simulink model "linear_system"  (R2021b)
settings: Solver=VariableStepAuto  StartTime=0.0  StopTime=10.0  RelTol=1e-8
values from neighbouring files (symbols this model uses):
  A = [ ... (first row only)    [linearized_model.m]
  B = [0; 0; c*F/E; b*F/E]    [linearized_model.m]
  C = [ ... (first row only)    [linearized_model.m]
  D = [0; 0]    [linearized_model.m]
undefined symbols (not defined in the file or in its folder): K
libraries: simulink_extras x2, simulink x2
settings Model: Creator=viking  LastModifiedBy=viking
settings SolverCC: ZeroCrossAlgorithm=Adaptive
settings DebuggingCC: UnconnectedInputMsg=none  UnconnectedOutputMsg=none  UnconnectedLineMsg=none
settings ModelReferenceCC: EnableRefExpFcnMdlSchedulingChecks=off
settings RTWCC: DLArmComputeVersion=20.02.1

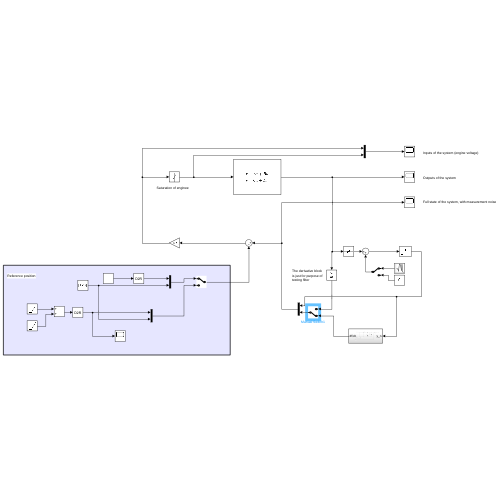
[thumbnail: Simulink's stored preview of the top-level diagram]
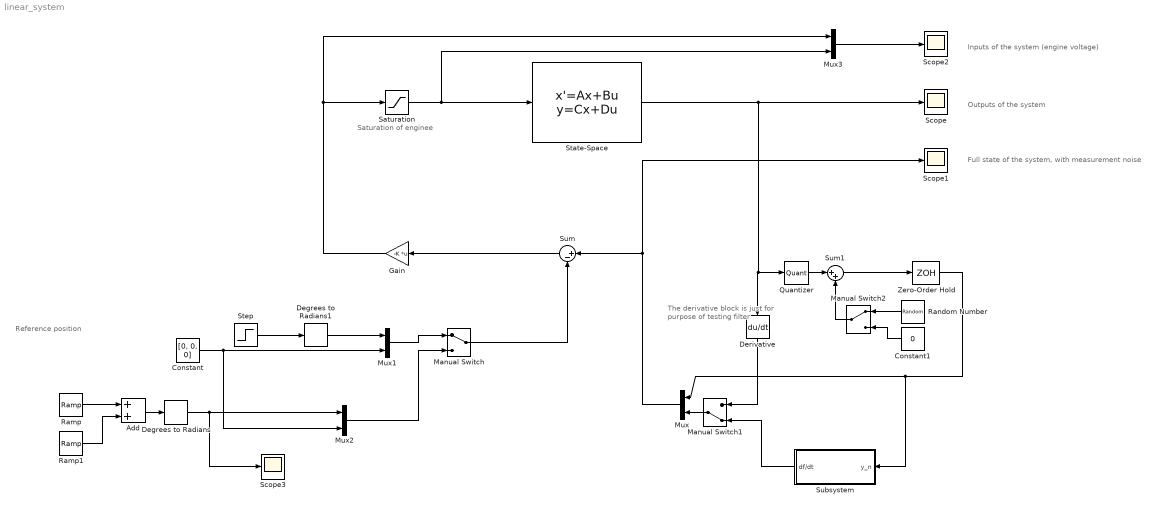
== system linear_system ==
  note: The derivative block is just for purpose of testing filter
  note: Inputs of the system (engine voltage)
  note: Full state of the system, with measurement noise
  note: Outputs of the system
  note: Saturation of enginee
  note: Reference position
  Add : Sum
  Constant : Constant  Value=[0, 0, 0]
  Constant1 : Constant  Value=0
  Degrees to Radians : simulink_extras/Transformations/Degrees to Radians
  Degrees to Radians1 : simulink_extras/Transformations/Degrees to Radians
  Derivative : Derivative  CoefficientInTFapproximation=0
  Gain : Gain  Gain=-K  Multiplication=Matrix(K*u)
  Manual Switch : ManualSwitch
  Manual Switch1 : ManualSwitch  CurrentSetting=0
  Manual Switch2 : ManualSwitch
  Mux{,1..3} (4 alike) : Mux  Inputs=2
  Quantizer : Quantizer  QuantizationInterval=0.005
  Ramp : simulink/Sources/Ramp  slope=5  start=0  InitialOutput=0
  Ramp1 : simulink/Sources/Ramp  slope=-5  start=5  InitialOutput=0
  Random Number : RandomNumber  Variance=1e-5  SampleTime=0.005
  Saturation : Saturate  UpperLimit=5  LowerLimit=-5
  Scope{,1..3} (4 alike) : Scope
  State-Space : StateSpace  A=A  B=B  C=C  D=D  InitialCondition=[0, 0, 0, 0]  ContinuousStateAttributes={'theta', 'alpha', 'dtheta', 'dalpha'}
  Step : Step  Time=0.1  After=45  SampleTime=0
  Subsystem : Subsystem
  Sum : Sum  Inputs=|+-
  Sum1 : Sum  Inputs=|++
  Zero-Order Hold : ZeroOrderHold  SampleTime=0.005
  wires:
  State-Space/1 -> Quantizer/1, Derivative/1, Scope/1
  Gain/1 -> Mux3/1, Saturation/1
  Mux/1 -> Sum/1, Scope1/1
  Sum/1 -> Gain/1
  Manual Switch/1 -> Sum/2
  Mux1/1 -> Manual Switch/1
  Constant/1 -> Mux2/2, Mux1/2
  Mux2/1 -> Manual Switch/2
  Ramp/1 -> Add/1
  Ramp1/1 -> Add/2
  Saturation/1 -> Mux3/2, State-Space/1
  Derivative/1 -> Manual Switch1/1
  Manual Switch1/1 -> Mux/2
  Subsystem/1(df/dt) -> Manual Switch1/2
  Degrees to Radians1/1 -> Mux1/1
  Step/1 -> Degrees to Radians1/1
  Add/1 -> Degrees to Radians/1
  Degrees to Radians/1 -> Scope3/1, Mux2/1
  Sum1/1 -> Zero-Order Hold/1
  Mux3/1 -> Scope2/1
  Quantizer/1 -> Sum1/1
  Zero-Order Hold/1 -> Subsystem/1(y_n), Mux/1
  Manual Switch2/1 -> Sum1/2
  Random Number/1 -> Manual Switch2/1
  Constant1/1 -> Manual Switch2/2

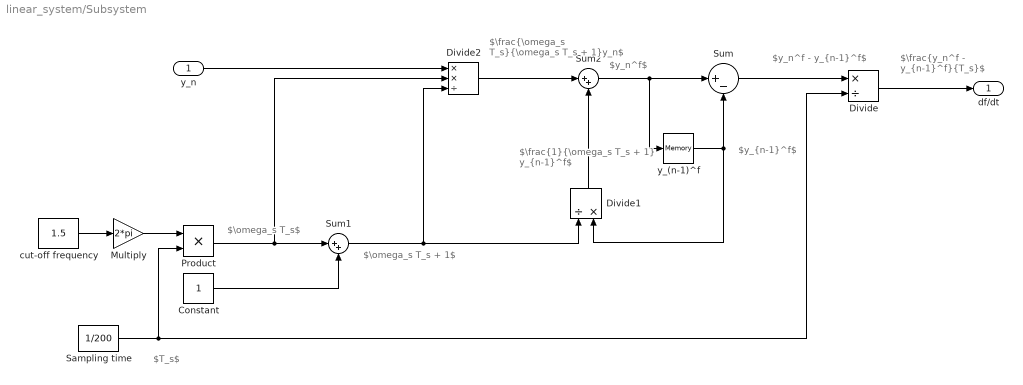
== system linear_system/Subsystem ==
  note: $\frac{y_n^f - y_{n-1}^f}{T_s}$
  note: $T_s$
  note: $y_n^f - y_{n-1}^f$
  note: $\frac{1}{\omega_s T_s + 1} y_{n-1}^f$
  note: $y_n^f$
  note: $y_{n-1}^f$
  note: $\frac{\omega_s T_s}{\omega_s T_s + 1}y_n$
  note: $\omega_s T_s$
  note: $\omega_s T_s + 1$
  y_n : Inport
  Constant : Constant
  Divide : Product  Inputs=*/
  Divide1 : Product  Inputs=/*
  Divide2 : Product  Inputs=**/
  Multiply : Gain  Gain=2*pi
  Product : Product
  Sampling time : Constant  Value=1/200
  Sum : Sum  Inputs=|+-
  Sum1 : Sum  Inputs=|++
  Sum2 : Sum  Inputs=|++
  cut-off frequency : Constant  Value=1.5
  y_(n-1)^f : Memory
  df/dt : Outport
  wires:
  Multiply/1 -> Product/1
  Sampling time/1 -> Product/2, Divide/2
  Product/1 -> Divide2/2, Sum1/1
  Sum1/1 -> Divide2/3, Divide1/1
  Constant/1 -> Sum1/2
  y_n/1 -> Divide2/1
  y_(n-1)^f/1 -> Divide1/2, Sum/2
  Sum/1 -> Divide/1
  Divide/1 -> df/dt/1
  Divide2/1 -> Sum2/1
  Sum2/1 -> y_(n-1)^f/1, Sum/1
  Divide1/1 -> Sum2/2
  cut-off frequency/1 -> Multiply/1
